simulink model "starshotsimv4p3lqrforautocode"  (R2017a)
settings: Solver=FixedStepAuto  StartTime=0.0  StopTime=1000  FixedStep=.01  MaxStep=4.0  MinStep=.001  RelTol=1e-6
values from neighbouring files (symbols this model uses):
  B0 = 3.12e-5    (= 3.12e-05)    [starshot_DC_KD_setupv2.m]    (also in starshot_IC_initv2.m)
  G = 6.67e-11    [starshot_DC_KD_setupv2.m]    (also in starshot_IC_initv2.m)
  M_Earth = 5.972e24    (= 5.972e+24)    [starshot_DC_KD_setupv2.m]    (also in starshot_IC_initv2.m)
  q0 = [qmatlab(2:4),qmatlab(1)]'    [starshot_DC_KD_setupv2.m]    (also in starshot_IC_initv2.m)
  R_Earth = 6.378e6    (= 6378000)    [starshot_DC_KD_setupv2.m]    (also in starshot_IC_initv2.m)
undefined symbols (not defined in the file or in its folder): DiscIntNeverNeededParam, starshot
libraries: vrlib x2, simulink x2, dspmathops x1
settings Model: Creator=armen  LastModifiedBy=armen
settings OptimizationCC: DefaultParameterBehavior=Inlined  UseDivisionForNetSlopeComputation=on  UseFloatMulNetSlope=on  InlineInvariantSignals=on  EnhancedBackFolding=on  BooleansAsBitfields=on  PassReuseOutputArgsAs=Individual arguments  StateBitsets=on  DataBitsets=on  ZeroExternalMemoryAtStartup=off  ZeroInternalMemoryAtStartup=off  NoFixptDivByZeroProtection=on  EfficientFloat2IntCast=on  LifeSpan=1
settings DebuggingCC: ParameterTunabilityLossMsg=error
settings HardwareCC: ProdBitPerPointer=32  ProdBitPerSizeT=32  ProdBitPerPtrDiffT=32  ProdLargestAtomicInteger=Long  ProdLargestAtomicFloat=Double  ProdWordSize=32  ProdHWDeviceType=ARM Compatible->ARM Cortex
settings SFSimCC: MATLABDynamicMemAlloc=off
settings RTWCC: SystemTargetFile=ert.tlc  TemplateMakefile=ert_default_tmf  Description=Embedded Coder  GenerateReport=on  IncludeHyperlinkInReport=on  LaunchReport=on  TargetLang=C++  GenerateTraceInfo=on  GenerateTraceReport=on  GenerateTraceReportSl=on  GenerateTraceReportSf=on  GenerateTraceReportEml=on
settings CodeAppCC: ForceParamTrailComments=on  IgnoreCustomStorageClasses=off  OperatorAnnotations=on  SimulinkDataObjDesc=on  SFDataObjDesc=on  MATLABFcnDesc=on  CustomSymbolStrGlobalVar=rt$N$M  CustomSymbolStrType=$N$M  CustomSymbolStrFcn=$N$M$F  CustomSymbolStrMacro=$N$M  InsertBlockDesc=on  MATLABSourceComments=on
settings ERTTargetCC: TargetLangStandard=C++03 (ISO)  GenerateSampleERTMain=on  IncludeMdlTerminateFcn=off  CombineSignalStateStructs=on  SuppressErrorStatus=on  SupportAbsoluteTime=off  MultiInstanceERTCode=on  CodeInterfacePackaging=C++ class  SupportComplex=off  InlinedParameterPlacement=NonHierarchical  RootIOFormat=Structure reference  ERTCustomFileTemplate=example_file_process.tlc  ERTFilePackagingFormat=CompactWithDataFile

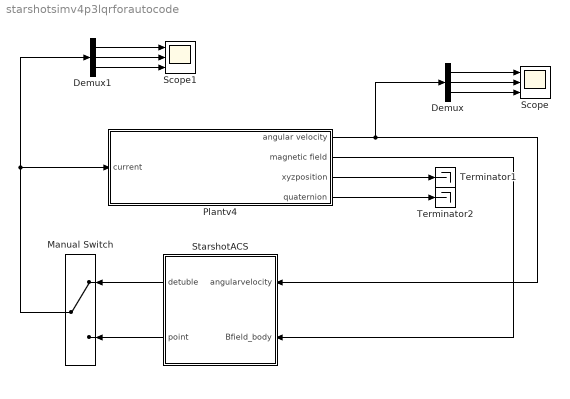
== system starshotsimv4p3lqrforautocode ==
  Demux : Demux  Outputs=3
  Demux1 : Demux  Outputs=3
  Manual Switch : ManualSwitch
  Plantv4 : Subsystem  TreatAsAtomicUnit=on
  Scope : Scope  NumInputPorts=3
  Scope1 : Scope  NumInputPorts=3
  StarshotACS : Subsystem  TreatAsAtomicUnit=on
  Terminator1 : Terminator
  Terminator2 : Terminator
  wires:
  Plantv4/2(magnetic field) -> StarshotACS/2(Bfield_body)
  Plantv4/1(angular velocity) -> Demux/1, StarshotACS/1(angularvelocity)
  Plantv4/3(xyzposition) -> Terminator1/1
  Plantv4/4(quaternion) -> Terminator2/1
  StarshotACS/2(point) -> Manual Switch/2
  StarshotACS/1(detuble) -> Manual Switch/1
  Demux/1 -> Scope/1
  Demux/2 -> Scope/2
  Demux/3 -> Scope/3
  Demux1/3 -> Scope1/3
  Demux1/2 -> Scope1/2
  Demux1/1 -> Scope1/1
  Manual Switch/1 -> Demux1/1, Plantv4/1(current)

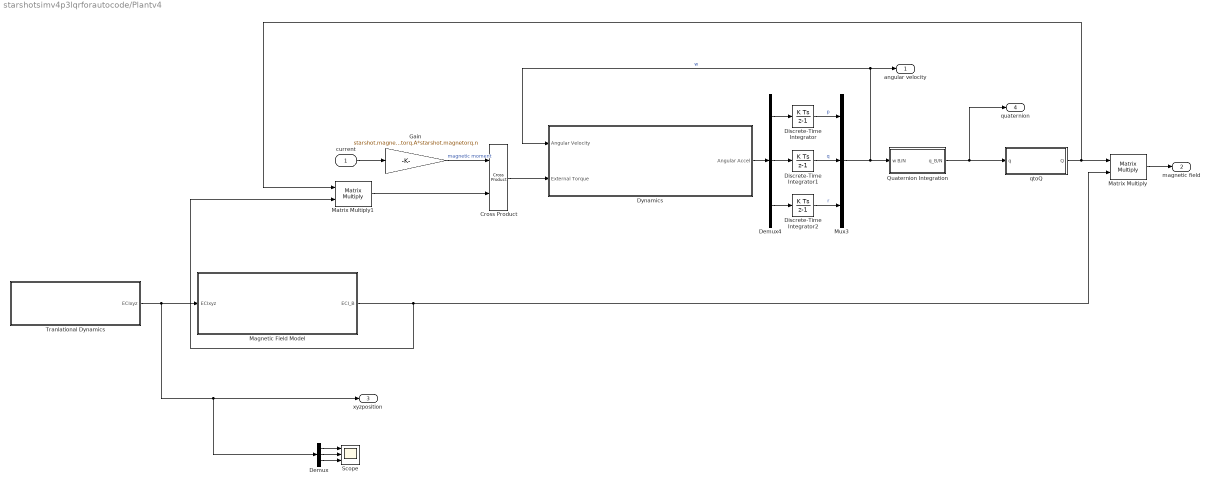
== system starshotsimv4p3lqrforautocode/Plantv4 ==
  current : Inport
  Cross Product : vrlib/Utilities/Cross Product
      settings: SourceProductBaseCode=VR
  Demux : Demux  Outputs=3
  Demux4 : Demux  Outputs=3
  Discrete-Time Integrator : DiscreteIntegrator  InitialCondition=starshot.IC.w(1)  InitialConditionSetting=State (most efficient)  SampleTime=-1  ICPrevOutput=DiscIntNeverNeededParam  ICPrevScaledInput=DiscIntNeverNeededParam
  Discrete-Time Integrator1 : DiscreteIntegrator  InitialCondition=starshot.IC.w(2)  InitialConditionSetting=State (most efficient)  SampleTime=-1  ICPrevOutput=DiscIntNeverNeededParam  ICPrevScaledInput=DiscIntNeverNeededParam
  Discrete-Time Integrator2 : DiscreteIntegrator  InitialCondition=starshot.IC.w(3)  InitialConditionSetting=State (most efficient)  SampleTime=-1  ICPrevOutput=DiscIntNeverNeededParam  ICPrevScaledInput=DiscIntNeverNeededParam
  Dynamics : Subsystem  TreatAsAtomicUnit=on
  Gain : Gain  Gain=starshot.magnetorq.A*starshot.magnetorq.n
  Magnetic Field Model : Subsystem  TreatAsAtomicUnit=on
  Matrix Multiply : Product  Multiplication=Matrix(*)
  Matrix Multiply1 : Product  Multiplication=Matrix(*)
  Mux3 : Mux  Inputs=3
  Quaternion Integration : Subsystem
  Scope : Scope  NumInputPorts=3
  Tranlational Dynamics : Subsystem  TreatAsAtomicUnit=on
  qtoQ : Subsystem  TreatAsAtomicUnit=on
  angular velocity : Outport
  magnetic field : Outport  Port=2
  xyzposition : Outport  Port=3
  quaternion : Outport  Port=4
  wires:
  Matrix Multiply/1 -> magnetic field/1
  Magnetic Field Model/1(ECI_B) -> Matrix Multiply1/2, Matrix Multiply/2
  Discrete-Time Integrator1/1 -> Mux3/2  "q"
  Discrete-Time Integrator2/1 -> Mux3/3  "r"
  Demux4/3 -> Discrete-Time Integrator2/1
  Demux4/1 -> Discrete-Time Integrator/1
  Tranlational Dynamics/1(ECIxyz) -> Demux/1, xyzposition/1, Magnetic Field Model/1(ECIxyz)
  Quaternion Integration/1(q_B/N) -> quaternion/1, qtoQ/1(q)
  Dynamics/1(Angular Accel) -> Demux4/1
  Mux3/1 -> Quaternion Integration/1(w B/N), Dynamics/1(Angular Velocity), angular velocity/1  "w"
  current/1 -> Gain/1
  Gain/1 -> Cross Product/1  "magnetic moment"
  Cross Product/1 -> Dynamics/2(External Torque)
  Discrete-Time Integrator/1 -> Mux3/1  "p"
  Demux4/2 -> Discrete-Time Integrator1/1
  Demux/2 -> Scope/2
  Demux/1 -> Scope/1
  Demux/3 -> Scope/3
  qtoQ/1(Q) -> Matrix Multiply1/1, Matrix Multiply/1
  Matrix Multiply1/1 -> Cross Product/2

== system starshotsimv4p3lqrforautocode/StarshotACS ==
  angularvelocity : Inport
  Bfield_body : Inport  Port=2
  KD_controller : Subsystem
  Orientation controller : Subsystem
  detuble : Outport
  point : Outport  Port=2
  wires:
  KD_controller/1(Dipole) -> detuble/1
  Orientation controller/1(Dipole) -> point/1
  Bfield_body/1 -> KD_controller/2(B(body)), Orientation controller/2(B(body))  "Bfield_body"
  angularvelocity/1 -> Orientation controller/1(Omega), KD_controller/1(Omega)  "angularvelocity"

== system starshotsimv4p3lqrforautocode/Plantv4/Dynamics ==
  Angular Velocity : Inport
  External Torque : Inport  Port=2
  Constant : Constant  Value=starshot.IC.massproperties.I
  Constant1 : Constant  Value=starshot.IC.massproperties.Iinv
  Cross Product : vrlib/Utilities/Cross Product
      settings: SourceProductBaseCode=VR
  Product : Product  Multiplication=Matrix(*)
  Product1 : Product  Multiplication=Matrix(*)
  Sum : Sum  Inputs=+-
  Angular Accel : Outport
  wires:
  Angular Velocity/1 -> Cross Product/1, Product/2
  Constant/1 -> Product/1
  Cross Product/1 -> Sum/2
  Product/1 -> Cross Product/2
  External Torque/1 -> Sum/1
  Constant1/1 -> Product1/1
  Product1/1 -> Angular Accel/1
  Sum/1 -> Product1/2

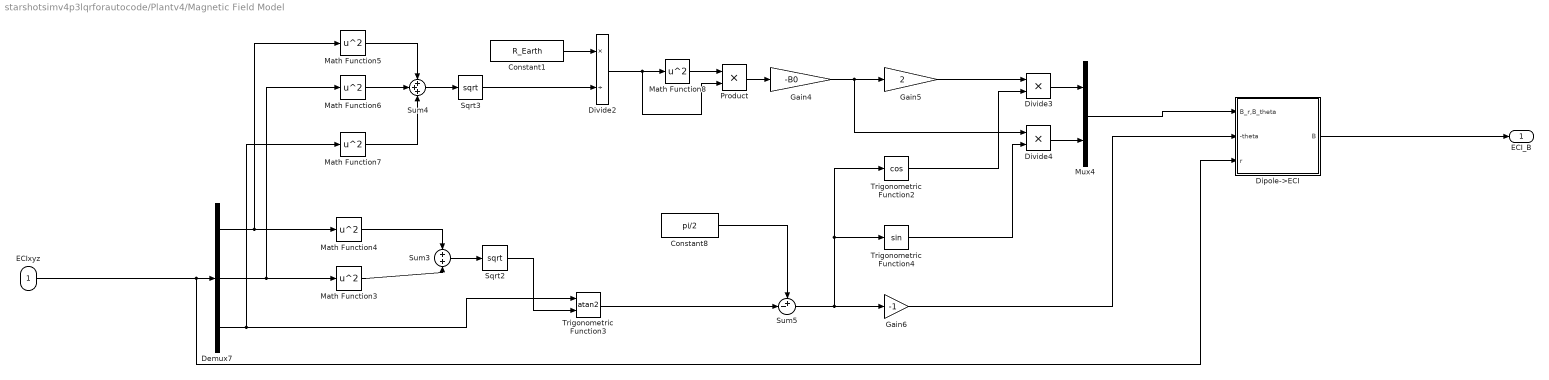
== system starshotsimv4p3lqrforautocode/Plantv4/Magnetic Field Model ==
  ECIxyz : Inport
  Constant1 : Constant  Value=R_Earth
  Constant8 : Constant  Value=pi/2
  Demux7 : Demux  Outputs=3
  Dipole->ECI : Subsystem  TreatAsAtomicUnit=on
  Divide2 : Product  Inputs=*/
  Divide3 : Product  Inputs=**
  Divide4 : Product  Inputs=**
  Gain4 : Gain  Gain=-B0
  Gain5 : Gain  Gain=2
  Gain6 : Gain  Gain=-1
  Math Function{3..8} (6 alike) : Math  Operator=square  SaturateOnIntegerOverflow=on
  Mux4 : Mux  Inputs=2
  Product : Product
  Sqrt2 : Sqrt  SaturateOnIntegerOverflow=on
  Sqrt3 : Sqrt  SaturateOnIntegerOverflow=on
  Sum3 : Sum
  Sum4 : Sum  Inputs=+++
  Sum5 : Sum  Inputs=+-|
  Trigonometric Function2 : Trigonometry  Operator=cos
  Trigonometric Function3 : Trigonometry  Operator=atan2
  Trigonometric Function4 : Trigonometry
  ECI_B : Outport
  wires:
  Math Function7/1 -> Sum4/3
  Constant1/1 -> Divide2/1
  Math Function5/1 -> Sum4/1
  Math Function4/1 -> Sum3/1
  Demux7/3 -> Math Function7/1, Trigonometric Function3/1
  Sqrt2/1 -> Trigonometric Function3/2
  Product/1 -> Gain4/1
  Math Function8/1 -> Product/1
  Gain5/1 -> Divide3/1
  Sqrt3/1 -> Divide2/2
  Sum4/1 -> Sqrt3/1
  Divide2/1 -> Product/2, Math Function8/1
  Sum3/1 -> Sqrt2/1
  Math Function3/1 -> Sum3/2
  Demux7/1 -> Math Function5/1, Math Function4/1
  Gain4/1 -> Gain5/1, Divide4/1
  Trigonometric Function2/1 -> Divide3/2
  Math Function6/1 -> Sum4/2
  Demux7/2 -> Math Function6/1, Math Function3/1
  Sum5/1 -> Trigonometric Function2/1, Trigonometric Function4/1, Gain6/1
  Trigonometric Function4/1 -> Divide4/2
  Gain6/1 -> Dipole->ECI/2(-theta)
  Divide4/1 -> Mux4/2
  Trigonometric Function3/1 -> Sum5/2
  Constant8/1 -> Sum5/1
  Mux4/1 -> Dipole->ECI/1(B_r,B_theta)
  Dipole->ECI/1(B) -> ECI_B/1
  Divide3/1 -> Mux4/1
  ECIxyz/1 -> Dipole->ECI/3(r), Demux7/1

== system starshotsimv4p3lqrforautocode/Plantv4/Quaternion Integration ==
  w B/N : Inport
  Discrete-Time Integrator1 : DiscreteIntegrator  InitialCondition=q0  InitialConditionSetting=State (most efficient)  SampleTime=-1  ICPrevOutput=DiscIntNeverNeededParam  ICPrevScaledInput=DiscIntNeverNeededParam
  q_normalize : Subsystem
  qderiv : Subsystem
  q_B/N : Outport
  wires:
  w B/N/1 -> qderiv/1(w)
  q_normalize/1(q_out) -> qderiv/2(q), q_B/N/1
  Discrete-Time Integrator1/1 -> q_normalize/1(q_in)
  qderiv/1(qd) -> Discrete-Time Integrator1/1

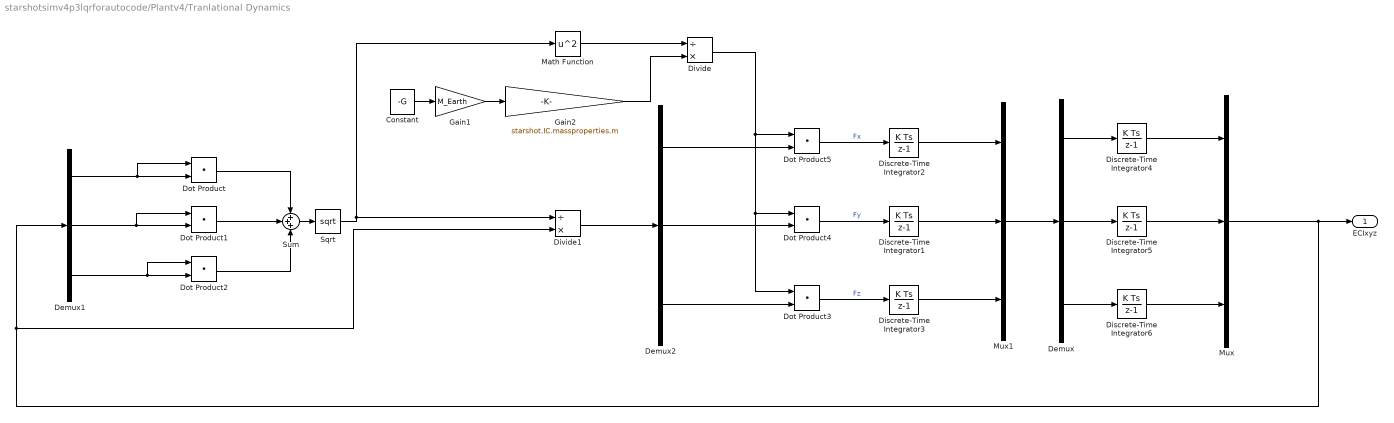
== system starshotsimv4p3lqrforautocode/Plantv4/Tranlational Dynamics ==
  Constant : Constant  Value=-G
  Demux : Demux  Outputs=3
  Demux1 : Demux  Outputs=3
  Demux2 : Demux  Outputs=3
  Discrete-Time Integrator1 : DiscreteIntegrator  InitialCondition=starshot.IC.ydot  InitialConditionSetting=State (most efficient)  SampleTime=-1  ICPrevOutput=DiscIntNeverNeededParam  ICPrevScaledInput=DiscIntNeverNeededParam
  Discrete-Time Integrator2 : DiscreteIntegrator  InitialCondition=starshot.IC.xdot  InitialConditionSetting=State (most efficient)  SampleTime=-1  ICPrevOutput=DiscIntNeverNeededParam  ICPrevScaledInput=DiscIntNeverNeededParam
  Discrete-Time Integrator3 : DiscreteIntegrator  InitialCondition=starshot.IC.zdot  InitialConditionSetting=State (most efficient)  SampleTime=-1  ICPrevOutput=DiscIntNeverNeededParam  ICPrevScaledInput=DiscIntNeverNeededParam
  Discrete-Time Integrator4 : DiscreteIntegrator  InitialCondition=starshot.IC.x  InitialConditionSetting=State (most efficient)  SampleTime=-1  ICPrevOutput=DiscIntNeverNeededParam  ICPrevScaledInput=DiscIntNeverNeededParam
  Discrete-Time Integrator5 : DiscreteIntegrator  InitialCondition=starshot.IC.y  InitialConditionSetting=State (most efficient)  SampleTime=-1  ICPrevOutput=DiscIntNeverNeededParam  ICPrevScaledInput=DiscIntNeverNeededParam
  Discrete-Time Integrator6 : DiscreteIntegrator  InitialCondition=starshot.IC.z  InitialConditionSetting=State (most efficient)  SampleTime=-1  ICPrevOutput=DiscIntNeverNeededParam  ICPrevScaledInput=DiscIntNeverNeededParam
  Divide : Product  Inputs=/*
  Divide1 : Product  Inputs=/*
  Dot Product{,1..5} (6 alike) : DotProduct  InputSameDT=on  OutDataTypeStr=Inherit: Inherit via internal rule
  Gain1 : Gain  Gain=M_Earth
  Gain2 : Gain  Gain=starshot.IC.massproperties.m
  Math Function : Math  Operator=square  SaturateOnIntegerOverflow=on
  Mux : Mux  Inputs=3
  Mux1 : Mux  Inputs=3
  Sqrt : Sqrt  SaturateOnIntegerOverflow=on
  Sum : Sum  Inputs=+++
  ECIxyz : Outport
  wires:
  Discrete-Time Integrator6/1 -> Mux/3
  Discrete-Time Integrator5/1 -> Mux/2
  Discrete-Time Integrator4/1 -> Mux/1
  Demux/3 -> Discrete-Time Integrator6/1
  Demux/1 -> Discrete-Time Integrator4/1
  Mux1/1 -> Demux/1
  Discrete-Time Integrator3/1 -> Mux1/3
  Demux/2 -> Discrete-Time Integrator5/1
  Demux1/2 -> Dot Product1/1, Dot Product1/2
  Sum/1 -> Sqrt/1
  Dot Product4/1 -> Discrete-Time Integrator1/1  "Fy"
  Demux1/1 -> Dot Product/1, Dot Product/2
  Dot Product3/1 -> Discrete-Time Integrator3/1  "Fz"
  Divide/1 -> Dot Product3/1, Dot Product4/1, Dot Product5/1
  Dot Product1/1 -> Sum/2
  Demux1/3 -> Dot Product2/1, Dot Product2/2
  Dot Product2/1 -> Sum/3
  Demux2/2 -> Dot Product4/2
  Demux2/3 -> Dot Product3/2
  Math Function/1 -> Divide/1
  Discrete-Time Integrator1/1 -> Mux1/2
  Gain1/1 -> Gain2/1
  Demux2/1 -> Dot Product5/2
  Dot Product5/1 -> Discrete-Time Integrator2/1  "Fx"
  Dot Product/1 -> Sum/1
  Constant/1 -> Gain1/1
  Divide1/1 -> Demux2/1
  Gain2/1 -> Divide/2
  Sqrt/1 -> Math Function/1, Divide1/1
  Discrete-Time Integrator2/1 -> Mux1/1
  Mux/1 -> ECIxyz/1, Divide1/2, Demux1/1

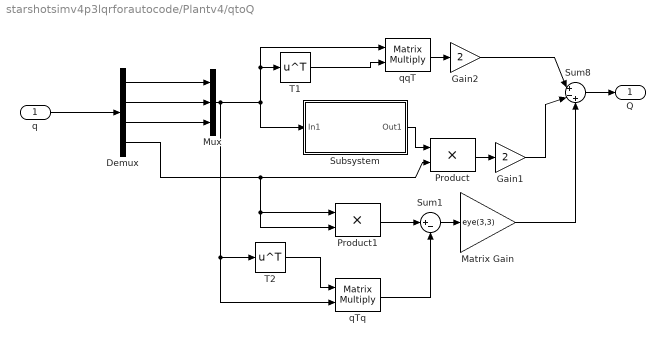
== system starshotsimv4p3lqrforautocode/Plantv4/qtoQ ==
  q : Inport
  Demux : Demux
  Gain1 : Gain  Gain=2  SaturateOnIntegerOverflow=on  OutDataTypeStr=Inherit: Same as input  ParamDataTypeStr=Inherit: Same as input
  Gain2 : Gain  Gain=2  SaturateOnIntegerOverflow=on  OutDataTypeStr=Inherit: Same as input  ParamDataTypeStr=Inherit: Same as input
  Matrix Gain : Gain  Gain=eye(3,3)  SaturateOnIntegerOverflow=on  OutDataTypeStr=Inherit: Same as input  ParamDataTypeStr=Inherit: Same as input
  Mux : Mux  Inputs=3
  Product : Product  SaturateOnIntegerOverflow=on  InputSameDT=on  OutDataTypeStr=Inherit: Same as first input
  Product1 : Product  SaturateOnIntegerOverflow=on  InputSameDT=on  OutDataTypeStr=Inherit: Same as first input
  Subsystem : Subsystem
      mask Display: disp('3x3 cross matrix')
  Sum1 : Sum  Inputs=|+-  SaturateOnIntegerOverflow=on  InputSameDT=on  OutDataTypeStr=Inherit: Same as first input
  Sum8 : Sum  Inputs=|+-+  SaturateOnIntegerOverflow=on  InputSameDT=on  OutDataTypeStr=Inherit: Same as first input
  T1 : Math  Operator=transpose  SaturateOnIntegerOverflow=on
  T2 : Math  Operator=transpose  SaturateOnIntegerOverflow=on
  qTq : Product  Multiplication=Matrix(*)  SaturateOnIntegerOverflow=on  InputSameDT=on  OutDataTypeStr=Inherit: Same as first input
  qqT : Product  Multiplication=Matrix(*)  SaturateOnIntegerOverflow=on  InputSameDT=on  OutDataTypeStr=Inherit: Same as first input
  Q : Outport
  wires:
  q/1 -> Demux/1
  Demux/1 -> Mux/1
  Matrix Gain/1 -> Sum8/3
  Demux/2 -> Mux/2
  Demux/3 -> Mux/3
  T2/1 -> qTq/1
  Demux/4 -> Product1/2, Product1/1, Product/2
  Product/1 -> Gain1/1
  qqT/1 -> Gain2/1
  Mux/1 -> qTq/2, T2/1, qqT/1, T1/1, Subsystem/1(In1)
  Sum8/1 -> Q/1
  Subsystem/1(Out1) -> Product/1
  Product1/1 -> Sum1/1
  Gain2/1 -> Sum8/1
  T1/1 -> qqT/2
  Gain1/1 -> Sum8/2
  qTq/1 -> Sum1/2
  Sum1/1 -> Matrix Gain/1

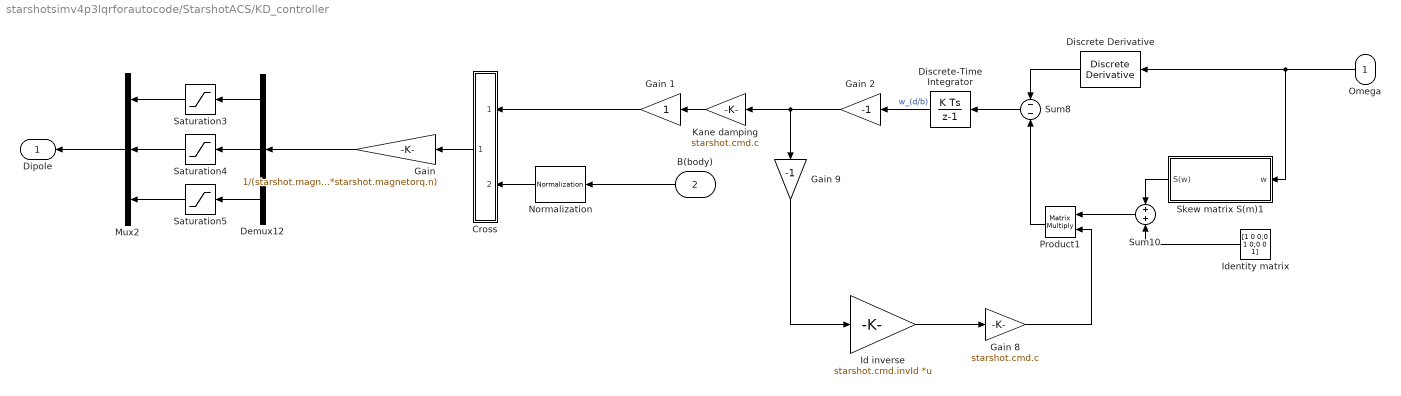
== system starshotsimv4p3lqrforautocode/StarshotACS/KD_controller ==
  Omega : Inport
  B(body) : Inport  Port=2
  Cross : Subsystem
  Demux12 : Demux  Outputs=3
  Discrete Derivative : simulink/Discrete/Discrete Derivative  gainval=1.0  ICPrevScaledInput=0.0  OutMin=[]  OutMax=[]  OutDataType=fixdt(1, 16)  OutScaling=2^-10  DoSatur=off
  Discrete-Time Integrator : DiscreteIntegrator  InitialCondition=starshot.cmd.wdb0  InitialConditionSetting=State (most efficient)  SampleTime=-1  ICPrevOutput=DiscIntNeverNeededParam  ICPrevScaledInput=DiscIntNeverNeededParam
  Gain : Gain  Gain=1/(starshot.magnetorq.A*starshot.magnetorq.n)
  Gain 1 : Gain  SaturateOnIntegerOverflow=on  OutDataTypeStr=Inherit: Same as input  ParamDataTypeStr=Inherit: Same as input
  Gain 2 : Gain  Gain=-1  SaturateOnIntegerOverflow=on  OutDataTypeStr=Inherit: Same as input  ParamDataTypeStr=Inherit: Same as input
  Gain 8 : Gain  Gain=starshot.cmd.c  SaturateOnIntegerOverflow=on  OutDataTypeStr=Inherit: Same as input  ParamDataTypeStr=Inherit: Same as input
  Gain 9 : Gain  Gain=-1  SaturateOnIntegerOverflow=on  OutDataTypeStr=Inherit: Same as input  ParamDataTypeStr=Inherit: Same as input
  Id inverse : Gain  Gain=starshot.cmd.invId  Multiplication=Matrix(K*u)  SaturateOnIntegerOverflow=on  OutDataTypeStr=Inherit: Same as input  ParamDataTypeStr=Inherit: Same as input
  Identity matrix : Constant  Value=[1 0 0;0 1 0;0 0 1]
  Kane damping : Gain  Gain=starshot.cmd.c  SaturateOnIntegerOverflow=on  OutDataTypeStr=Inherit: Same as input  ParamDataTypeStr=Inherit: Same as input
  Mux2 : Mux  Inputs=3
  Normalization : dspmathops/Normalization  NormType=Squared 2-norm  Bias=1e-10  NormOver=Each column  Dimension=1  outputDataTypeStr=Inherit: Same as product output  outputLastDataTypeStr=Inherit: Same as product output  outputMin=[]  outputMax=[]  accumDataTypeStr=Inherit: Same as product output  accumLastDataTypeStr=Inherit: Same as product output  roundingMode=Floor  overflowMode=off
      settings: SourceProductName=DSP System Toolbox
  Product1 : Product  Multiplication=Matrix(*)
  Saturation3 : Saturate  UpperLimit=starshot.magnetorq.m_max_x/(starshot.magnetorq.A*starshot.magnetorq.n)  LowerLimit=-starshot.magnetorq.m_max_x/(starshot.magnetorq.A*starshot.magnetorq.n)
  Saturation4 : Saturate  UpperLimit=starshot.magnetorq.m_max_y/(starshot.magnetorq.A*starshot.magnetorq.n)  LowerLimit=-starshot.magnetorq.m_max_y/(starshot.magnetorq.A*starshot.magnetorq.n)
  Saturation5 : Saturate  UpperLimit=starshot.magnetorq.m_max_z/(starshot.magnetorq.A*starshot.magnetorq.n)  LowerLimit=-starshot.magnetorq.m_max_z/(starshot.magnetorq.A*starshot.magnetorq.n)
  Skew matrix S(m)1 : Subsystem
  Sum10 : Sum  Inputs=+|+  SaturateOnIntegerOverflow=on  InputSameDT=on  OutDataTypeStr=Inherit: Same as first input
  Sum8 : Sum  Inputs=--
  Dipole : Outport
  wires:
  Discrete-Time Integrator/1 -> Gain 2/1  "w_(d/b)"
  Omega/1 -> Discrete Derivative/1, Skew matrix S(m)1/1(w)
  B(body)/1 -> Normalization/1
  Cross/1(AxB) -> Gain/1
  Gain 2/1 -> Kane damping/1, Gain 9/1
  Normalization/1 -> Cross/2(B)
  Kane damping/1 -> Gain 1/1
  Discrete Derivative/1 -> Sum8/1
  Sum8/1 -> Discrete-Time Integrator/1
  Gain 8/1 -> Product1/2
  Id inverse/1 -> Gain 8/1
  Skew matrix S(m)1/1(S(w)) -> Sum10/1
  Identity matrix/1 -> Sum10/2
  Gain 9/1 -> Id inverse/1
  Sum10/1 -> Product1/1
  Product1/1 -> Sum8/2
  Gain 1/1 -> Cross/1(A)
  Gain/1 -> Demux12/1
  Demux12/1 -> Saturation3/1
  Saturation3/1 -> Mux2/1
  Saturation5/1 -> Mux2/3
  Demux12/2 -> Saturation4/1
  Saturation4/1 -> Mux2/2
  Demux12/3 -> Saturation5/1
  Mux2/1 -> Dipole/1

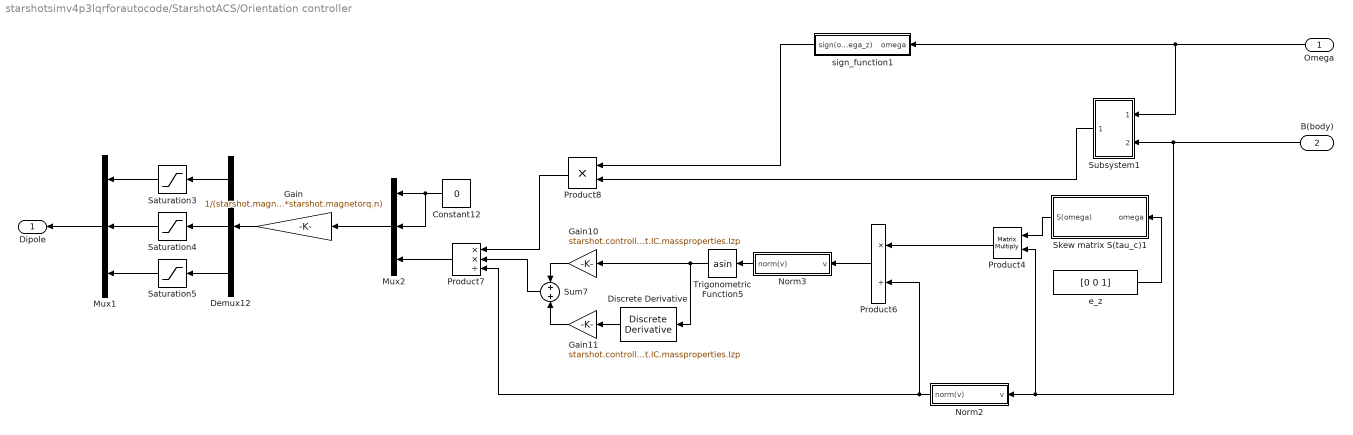
== system starshotsimv4p3lqrforautocode/StarshotACS/Orientation controller ==
  Omega : Inport
  B(body) : Inport  Port=2
  Constant12 : Constant  Value=0
  Demux12 : Demux  Outputs=3
  Discrete Derivative : simulink/Discrete/Discrete Derivative  gainval=1.0  ICPrevScaledInput=0.0  OutMin=[]  OutMax=[]  OutDataType=fixdt(1, 16)  OutScaling=2^-10  DoSatur=off
  Gain : Gain  Gain=1/(starshot.magnetorq.A*starshot.magnetorq.n)
  Gain10 : Gain  Gain=starshot.controller.Kp*starshot.IC.massproperties.Izp
  Gain11 : Gain  Gain=starshot.controller.Kd*starshot.IC.massproperties.Izp
  Mux1 : Mux  Inputs=3
  Mux2 : Mux  Inputs=3
  Norm2 : Subsystem
  Norm3 : Subsystem
  Product4 : Product  Multiplication=Matrix(*)
  Product6 : Product  Inputs=*/
  Product7 : Product  Inputs=**/
  Product8 : Product  Inputs=**
  Saturation3 : Saturate  UpperLimit=starshot.magnetorq.m_max_x/(starshot.magnetorq.A*starshot.magnetorq.n)  LowerLimit=-starshot.magnetorq.m_max_x/(starshot.magnetorq.A*starshot.magnetorq.n)
  Saturation4 : Saturate  UpperLimit=starshot.magnetorq.m_max_y/(starshot.magnetorq.A*starshot.magnetorq.n)  LowerLimit=-starshot.magnetorq.m_max_y/(starshot.magnetorq.A*starshot.magnetorq.n)
  Saturation5 : Saturate  UpperLimit=starshot.magnetorq.m_max_z/(starshot.magnetorq.A*starshot.magnetorq.n)  LowerLimit=-starshot.magnetorq.m_max_z/(starshot.magnetorq.A*starshot.magnetorq.n)
  Skew matrix S(tau_c)1 : Subsystem
  Subsystem1 : Subsystem
  Sum7 : Sum  Inputs=+|+
  Trigonometric Function5 : Trigonometry  Operator=asin
  e_z : Constant  Value=[0 0 1]
  sign_function1 : Subsystem
  Dipole : Outport
  wires:
  Product4/1 -> Product6/1
  Mux2/1 -> Gain/1
  Sum7/1 -> Product7/2
  Trigonometric Function5/1 -> Gain10/1, Discrete Derivative/1
  Norm3/1(norm(v)) -> Trigonometric Function5/1
  e_z/1 -> Skew matrix S(tau_c)1/1(omega)
  Product7/1 -> Mux2/3
  Constant12/1 -> Mux2/2, Mux2/1
  Skew matrix S(tau_c)1/1(S(omega)) -> Product4/1
  Discrete Derivative/1 -> Gain11/1
  Norm2/1(norm(v)) -> Product7/3, Product6/2
  Gain10/1 -> Sum7/1
  Product6/1 -> Norm3/1(v)
  Product8/1 -> Product7/1
  Gain11/1 -> Sum7/2
  B(body)/1 -> Product4/2, Norm2/1(v), Subsystem1/2(B(body))
  sign_function1/1(sign(omega_z)) -> Product8/1
  Subsystem1/1(sign(cos)) -> Product8/2
  Omega/1 -> Subsystem1/1(omega), sign_function1/1(omega)
  Gain/1 -> Demux12/1
  Demux12/1 -> Saturation3/1
  Saturation3/1 -> Mux1/1
  Saturation5/1 -> Mux1/3
  Demux12/2 -> Saturation4/1
  Saturation4/1 -> Mux1/2
  Demux12/3 -> Saturation5/1
  Mux1/1 -> Dipole/1

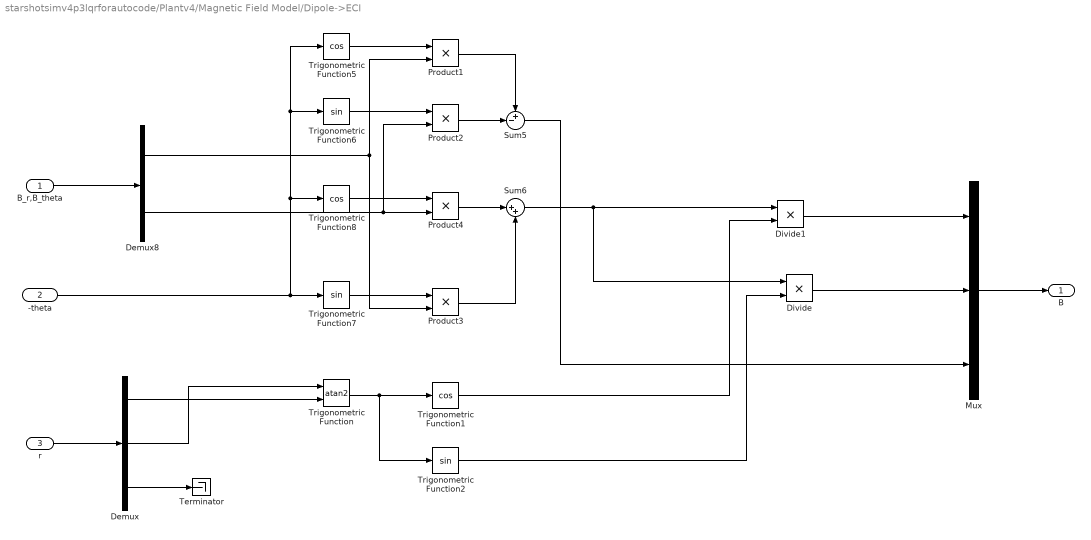
== system starshotsimv4p3lqrforautocode/Plantv4/Magnetic Field Model/Dipole->ECI ==
  B_r,B_theta : Inport
  -theta : Inport  Port=2
  r : Inport  Port=3
  Demux : Demux  Outputs=3
  Demux8 : Demux  Outputs=2
  Divide : Product  Inputs=**
  Divide1 : Product  Inputs=**
  Mux : Mux  Inputs=3
  Product{1..4} (4 alike) : Product
  Sum5 : Sum  Inputs=+-|
  Sum6 : Sum  Inputs=|++
  Terminator : Terminator
  Trigonometric Function : Trigonometry  Operator=atan2
  Trigonometric Function1 : Trigonometry  Operator=cos
  Trigonometric Function2 : Trigonometry
  Trigonometric Function5 : Trigonometry  Operator=cos
  Trigonometric Function6 : Trigonometry
  Trigonometric Function7 : Trigonometry
  Trigonometric Function8 : Trigonometry  Operator=cos
  B : Outport
  wires:
  -theta/1 -> Trigonometric Function5/1, Trigonometric Function6/1, Trigonometric Function8/1, Trigonometric Function7/1
  Product4/1 -> Sum6/1
  Product3/1 -> Sum6/2
  Demux8/1 -> Product3/2, Product1/2
  Demux8/2 -> Product2/2, Product4/2
  Trigonometric Function5/1 -> Product1/1
  Product2/1 -> Sum5/2
  Trigonometric Function7/1 -> Product3/1
  B_r,B_theta/1 -> Demux8/1
  Sum5/1 -> Mux/3
  Trigonometric Function8/1 -> Product4/1
  Trigonometric Function6/1 -> Product2/1
  Sum6/1 -> Divide1/1, Divide/1
  Product1/1 -> Sum5/1
  r/1 -> Demux/1
  Demux/3 -> Terminator/1
  Demux/2 -> Trigonometric Function/1
  Demux/1 -> Trigonometric Function/2
  Trigonometric Function/1 -> Trigonometric Function1/1, Trigonometric Function2/1
  Trigonometric Function1/1 -> Divide1/2
  Trigonometric Function2/1 -> Divide/2
  Mux/1 -> B/1
  Divide1/1 -> Mux/1
  Divide/1 -> Mux/2

== system starshotsimv4p3lqrforautocode/Plantv4/Quaternion Integration/q_normalize ==
  q_in : Inport  PortDimensions=4
  Dot Product : DotProduct  InputSameDT=on  OutDataTypeStr=Inherit: Inherit via internal rule
  Math Function : Math  Operator=sqrt  SaturateOnIntegerOverflow=on
  Product : Product  Inputs=*/  SaturateOnIntegerOverflow=on  InputSameDT=on  OutDataTypeStr=Inherit: Same as first input
  q_out : Outport
  wires:
  Product/1 -> q_out/1
  Math Function/1 -> Product/2
  Dot Product/1 -> Math Function/1
  q_in/1 -> Dot Product/2, Dot Product/1, Product/1

== system starshotsimv4p3lqrforautocode/Plantv4/Quaternion Integration/qderiv ==
  w : Inport
  q : Inport  Port=2
  Mux : Mux  Inputs=2
  Mux1 : Mux
  qd1 : Fcn  Expr=(u(7)*u(1)-u(6)*u(2)+u(5)*u(3))/2
  qd2 : Fcn  Expr=(u(6)*u(1)+u(7)*u(2)-u(4)*u(3))/2
  qd3 : Fcn  Expr=(-u(5)*u(1)+u(4)*u(2)+u(7)*u(3))/2
  qd4 : Fcn  Expr=(-u(4)*u(1)-u(5)*u(2)-u(6)*u(3))/2
  qd : Outport
  wires:
  Mux1/1 -> qd/1
  qd4/1 -> Mux1/4
  qd3/1 -> Mux1/3
  qd2/1 -> Mux1/2
  qd1/1 -> Mux1/1
  Mux/1 -> qd4/1, qd3/1, qd2/1, qd1/1
  q/1 -> Mux/2
  w/1 -> Mux/1

== system starshotsimv4p3lqrforautocode/Plantv4/qtoQ/Subsystem ==
  In1 : Inport
  3x3 : Reshape  OutputDimensionality=Customize  OutputDimensions=[3,3]
  Demux : Demux  Outputs=3
  Gain : Gain  Gain=-1  SaturateOnIntegerOverflow=on  OutDataTypeStr=Inherit: Same as input  ParamDataTypeStr=Inherit: Same as input
  Gain1 : Gain  Gain=-1  SaturateOnIntegerOverflow=on  OutDataTypeStr=Inherit: Same as input  ParamDataTypeStr=Inherit: Same as input
  Gain2 : Gain  Gain=-1  SaturateOnIntegerOverflow=on  OutDataTypeStr=Inherit: Same as input  ParamDataTypeStr=Inherit: Same as input
  Mux : Mux  Inputs=9
  "diag 0 " : Constant  Value=0
  Out1 : Outport
  wires:
  Gain2/1 -> Mux/8
  Demux/1 -> Gain2/1, Mux/6
  Gain1/1 -> Mux/4
  Demux/2 -> Mux/7, Gain/1
  Gain/1 -> Mux/3
  Demux/3 -> Gain1/1, Mux/2
  Mux/1 -> 3x3/1
  "diag 0 "/1 -> Mux/9, Mux/5, Mux/1
  3x3/1 -> Out1/1
  In1/1 -> Demux/1

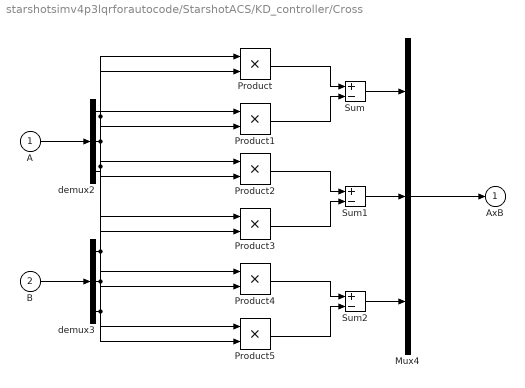
== system starshotsimv4p3lqrforautocode/StarshotACS/KD_controller/Cross ==
  A : Inport
  B : Inport  Port=2
  Mux4 : Mux  Inputs=3
  Product{,1..5} (6 alike) : Product  SaturateOnIntegerOverflow=on  InputSameDT=on  OutDataTypeStr=Inherit: Same as first input
  Sum : Sum  Inputs=+-  SaturateOnIntegerOverflow=on  InputSameDT=on  OutDataTypeStr=Inherit: Same as first input
  Sum1 : Sum  Inputs=+-  SaturateOnIntegerOverflow=on  InputSameDT=on  OutDataTypeStr=Inherit: Same as first input
  Sum2 : Sum  Inputs=+-  SaturateOnIntegerOverflow=on  InputSameDT=on  OutDataTypeStr=Inherit: Same as first input
  demux2 : Demux  Outputs=3
  demux3 : Demux  Outputs=3
  AxB : Outport  InitialOutput=0
  wires:
  A/1 -> demux2/1
  B/1 -> demux3/1
  demux2/3 -> Product1/1, Product2/1
  demux3/3 -> Product/2, Product3/2
  demux2/1 -> Product3/1, Product4/1
  demux3/2 -> Product1/2, Product4/2
  demux2/2 -> Product/1, Product5/1
  demux3/1 -> Product2/2, Product5/2
  Product/1 -> Sum/1
  Product1/1 -> Sum/2
  Product2/1 -> Sum1/1
  Product3/1 -> Sum1/2
  Product4/1 -> Sum2/1
  Product5/1 -> Sum2/2
  Sum/1 -> Mux4/1
  Sum1/1 -> Mux4/2
  Sum2/1 -> Mux4/3
  Mux4/1 -> AxB/1

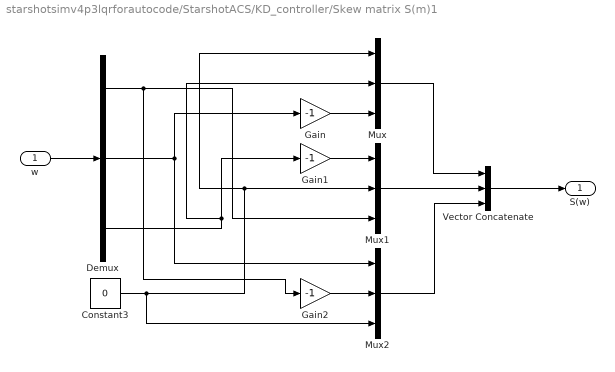
== system starshotsimv4p3lqrforautocode/StarshotACS/KD_controller/Skew matrix S(m)1 ==
  w : Inport
  Constant3 : Constant  Value=0
  Demux : Demux  Outputs=3
  Gain : Gain  Gain=-1
  Gain1 : Gain  Gain=-1
  Gain2 : Gain  Gain=-1
  Mux : Mux  Inputs=3
  Mux1 : Mux  Inputs=3
  Mux2 : Mux  Inputs=3
  Vector Concatenate : Concatenate  NumInputs=3  Mode=Multidimensional array  ConcatenateDimension=2
  S(w) : Outport
  wires:
  Gain/1 -> Mux/3
  Demux/2 -> Mux2/1, Gain/1
  Demux/3 -> Gain1/1, Mux/2
  Gain2/1 -> Mux2/2
  Demux/1 -> Mux1/3, Gain2/1
  Mux1/1 -> Vector Concatenate/2
  w/1 -> Demux/1
  Constant3/1 -> Mux2/3, Mux/1, Mux1/2
  Vector Concatenate/1 -> S(w)/1
  Mux/1 -> Vector Concatenate/1
  Mux2/1 -> Vector Concatenate/3
  Gain1/1 -> Mux1/1

== system starshotsimv4p3lqrforautocode/StarshotACS/Orientation controller/Norm2 ==
  v : Inport
  Dot Product6 : DotProduct  InputSameDT=on  OutDataTypeStr=Inherit: Inherit via internal rule
  Sqrt4 : Sqrt  SaturateOnIntegerOverflow=on
  norm(v) : Outport
  wires:
  v/1 -> Dot Product6/1, Dot Product6/2
  Dot Product6/1 -> Sqrt4/1
  Sqrt4/1 -> norm(v)/1

== system starshotsimv4p3lqrforautocode/StarshotACS/Orientation controller/Norm3 ==
  v : Inport
  Dot Product6 : DotProduct  InputSameDT=on  OutDataTypeStr=Inherit: Inherit via internal rule
  Sqrt4 : Sqrt  SaturateOnIntegerOverflow=on
  norm(v) : Outport
  wires:
  v/1 -> Dot Product6/1, Dot Product6/2
  Dot Product6/1 -> Sqrt4/1
  Sqrt4/1 -> norm(v)/1

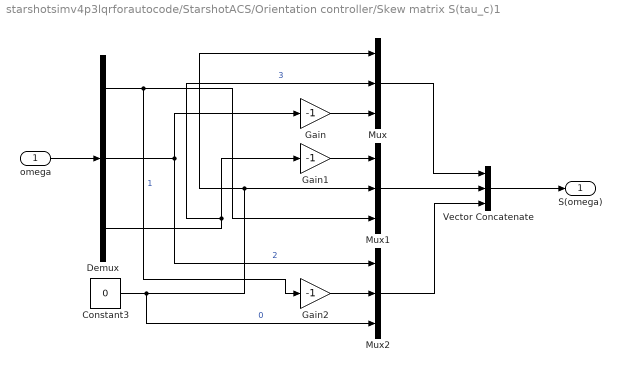
== system starshotsimv4p3lqrforautocode/StarshotACS/Orientation controller/Skew matrix S(tau_c)1 ==
  omega : Inport
  Constant3 : Constant  Value=0
  Demux : Demux  Outputs=3
  Gain : Gain  Gain=-1
  Gain1 : Gain  Gain=-1
  Gain2 : Gain  Gain=-1
  Mux : Mux  Inputs=3
  Mux1 : Mux  Inputs=3
  Mux2 : Mux  Inputs=3
  Vector Concatenate : Concatenate  NumInputs=3  Mode=Multidimensional array  ConcatenateDimension=2
  S(omega) : Outport
  wires:
  Gain/1 -> Mux/3
  Demux/2 -> Mux2/1, Gain/1  "2"
  Demux/3 -> Gain1/1, Mux/2  "3"
  Gain2/1 -> Mux2/2
  Demux/1 -> Mux1/3, Gain2/1  "1"
  Mux1/1 -> Vector Concatenate/2
  omega/1 -> Demux/1
  Constant3/1 -> Mux2/3, Mux/1, Mux1/2  "0"
  Vector Concatenate/1 -> S(omega)/1
  Mux/1 -> Vector Concatenate/1
  Mux2/1 -> Vector Concatenate/3
  Gain1/1 -> Mux1/1

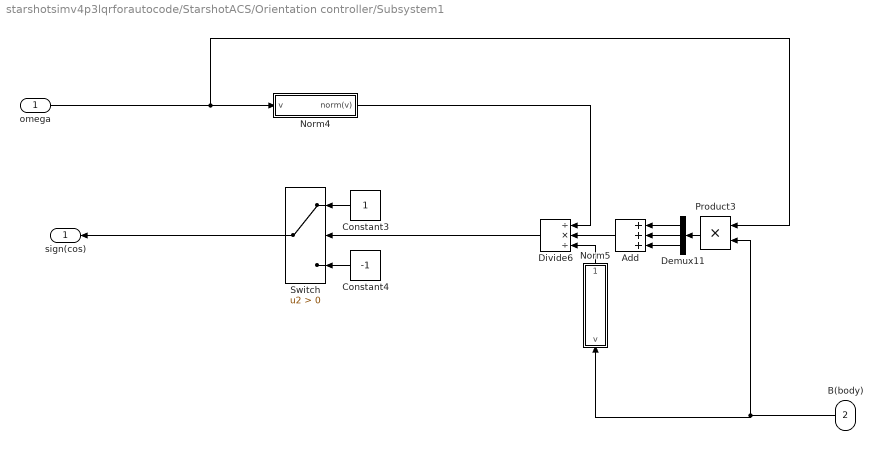
== system starshotsimv4p3lqrforautocode/StarshotACS/Orientation controller/Subsystem1 ==
  omega : Inport
  B(body) : Inport  Port=2
  Add : Sum  Inputs=3
  Constant3 : Constant
  Constant4 : Constant  Value=-1
  Demux11 : Demux  Outputs=3
  Divide6 : Product  Inputs=/*/
  Norm4 : Subsystem
  Norm5 : Subsystem
  Product3 : Product
  Switch : Switch  Criteria=u2 > Threshold  ZeroCross=off
  sign(cos) : Outport
  wires:
  Switch/1 -> sign(cos)/1
  Constant4/1 -> Switch/3
  Add/1 -> Divide6/2
  Constant3/1 -> Switch/1
  Demux11/3 -> Add/3
  Norm4/1(norm(v)) -> Divide6/1
  Divide6/1 -> Switch/2
  Norm5/1(norm(v)) -> Divide6/3
  Product3/1 -> Demux11/1
  Demux11/1 -> Add/1
  Demux11/2 -> Add/2
  B(body)/1 -> Norm5/1(v), Product3/2
  omega/1 -> Product3/1, Norm4/1(v)

== system starshotsimv4p3lqrforautocode/StarshotACS/Orientation controller/sign_function1 ==
  omega : Inport
  Constant10 : Constant  Value=-1
  Constant9 : Constant
  Selector : Selector  InputPortWidth=3  IndexOptions=Index vector (dialog)  Indices=[3]  OutputSizes=1
  Switch1 : Switch  ZeroCross=off
  sign(omega_z) : Outport
  wires:
  Constant9/1 -> Switch1/1
  Constant10/1 -> Switch1/3
  Switch1/1 -> sign(omega_z)/1
  Selector/1 -> Switch1/2
  omega/1 -> Selector/1

== system starshotsimv4p3lqrforautocode/StarshotACS/Orientation controller/Subsystem1/Norm4 ==
  v : Inport
  Dot Product6 : DotProduct  InputSameDT=on  OutDataTypeStr=Inherit: Inherit via internal rule
  Sqrt4 : Sqrt  SaturateOnIntegerOverflow=on
  norm(v) : Outport
  wires:
  v/1 -> Dot Product6/1, Dot Product6/2
  Dot Product6/1 -> Sqrt4/1
  Sqrt4/1 -> norm(v)/1

== system starshotsimv4p3lqrforautocode/StarshotACS/Orientation controller/Subsystem1/Norm5 ==
  v : Inport
  Dot Product6 : DotProduct  InputSameDT=on  OutDataTypeStr=Inherit: Inherit via internal rule
  Sqrt4 : Sqrt  SaturateOnIntegerOverflow=on
  norm(v) : Outport
  wires:
  v/1 -> Dot Product6/1, Dot Product6/2
  Dot Product6/1 -> Sqrt4/1
  Sqrt4/1 -> norm(v)/1
